simulink model "OBJMIL"  (Simulink 8.2)
settings: Solver=FixedStepDiscrete  StartTime=0.0  StopTime=126  FixedStep=0.005  RelTol=1e-3
PostLoadFcn:
  | , if any(exist('dsrtsu_mdlpostloadfcn', 'file') == [2, 3, 6]), try dsrtsu_mdlpostloadfcn('Execute', bdroot); catch fprintf('Error in PostLoadFcn (dsrtsu_mdlpostloadfcn) for model "%s":\n %s\n', bdroot, lasterr); end, end,
values from neighbouring files (symbols this model uses):
  C_TASK_5MS_S = (	C_TICK_TIME_S      	)    [hcu_local_hdr.m]
  ENUM_GEARPOSN_1ST = uint8(  1  )    [hcu_local_hdr.m]
  ENUM_GEARPOSN_R = uint8(  7  )    [hcu_local_hdr.m]
  FALSE = boolean( 0 )    [hcu_local_hdr.m]
  R_OBJ_Position = single([ii 0 0])    [GridSearch.m]
  R_OBJ_RelAccel = single([0 0 kk])    [GridSearch.m]
  R_OBJ_RelVelocity = single([0 jj 0])    [GridSearch.m]
  TRUE = boolean( 1 )    [hcu_local_hdr.m]
undefined symbols (not defined in the file or in its folder): A_OBJ, B_OBJ, C_OBJ, Gamma_OBJ, KOBJ_KalmanFilterCalRate_s, KOBJ_UseCalObjSpd_flg, KOBJ_UseEstObjInfo_flg, KOBJ_VehAccCalRate_s, KOBJ_VehAccFltConst_s, Q_OBJ, slcm
libraries: simulink x39, hcu_lib x10, dspmtrx3 x3, dspinverses x1
(part 1 of 2)
settings Model: DSRTSU_INTERNAL_RTI_VER=460  DSRTSU_INTERNAL_RTI_TYPE=rti1401  RTICANMMDATA=struct('GeneralSetupData',struct('modelroot','D:\HAITEC\SVN\trunk\ADAS_Softwares\HTDragon\software\sw_development\arch','generalsettings',struct('filesettings',struct('destfolder',struct('Name','RTICANMM_FILES','Check',1),'buildfolder',struct('Name','.','Check',1),'AbsDestfolder',struct('Name','D:\HAITEC\SVN\trunk\ADAS_Softwares\HTDragon\software\sw_development\arch\RTICANMM_FILES'),'AbsBuildfolder',struct('Name','D:\HAITEC\SVN\trunk\ADAS_Softwares\HTDragon\software\sw_development\arch'))),'options',struct('addpaths',1,'rmpaths',1,'addtrcexclusion',logical(1),'cannavigator',struct('checkmonitoring',0),'show_usrtrc',0,'use_usrtrc',0),'advanced',struct('options',[1 1 1 1 1 1 1 1 1 1 1 1 1 1 1 1 1 1 1 1 1 1 1 1 1 1 1 1 1 1 1 1 1 1 1 1 1 1 1 1 1 1 1 1 1 1 1 1 1 1 1 1 1 1 1 1 1 1 1 1 1 1 1 1 1 1 1 1 1 1 1 1 1 1 1 1 1 1 1 1 1 1 1 1 1 1 1 1 1 1 1 1 1 1 1 1 1 1 1 1]),'MPSetup',{{}},'modelname','OBJMIL','block','OBJMIL'))  DSRTSU_INTERNAL_RTIFPGA=50  Creator=14014  LastModifiedBy=14014  BufferReuse=off
settings DataIOCC: SignalLoggingSaveFormat=Dataset
settings OptimizationCC: BlockReduction=off  OptimizeBlockIOStorage=off  BufferReuse=off  ExpressionFolding=off  ExpressionDepthLimit=128  LocalBlockOutputs=off
settings DebuggingCC: ParameterPrecisionLossMsg=none  FcnCallInpInsideContextMsg=EnableAllAsError  StateNameClashWarn=none
settings HardwareCC: ProdIntDivRoundTo=Zero  ProdEndianess=BigEndian  ProdHWDeviceType=Generic->Custom  TargetIntDivRoundTo=Zero  TargetEndianess=BigEndian  TargetHWDeviceType=Generic->Custom
settings RTWCC: SystemTargetFile=rti1401.tlc  MakeCommand=make_rti  TemplateMakefile=rti1401.tmf  Description=dSPACE DS1401 Hardware Platform  ProcessScript=rti1401_make_rtw_hook
settings STFCustomTargetCC: CodeReplacementLibrary=ANSI_C  ParMdlRefBuildCompliant=on  GeneratePreprocessorConditionals=Disable all  MatFileLogging=on  SystemTargetFile=rti1401.tlc
settings GRTTargetCC: CompOptLevelCompliant=off  ConcurrentExecutionCompliant=off  ExtModeMexFile=noextcomm
settings CustomProperty: DataType=RTWOptions_EnumType_C__Program Files_dSPACE RCPHIL 2015-A_MATLAB_RTI_RTI1401_TLC_rti1401_1InitialSimState  Value=RUN
settings EnumStrPairs: String=RUN

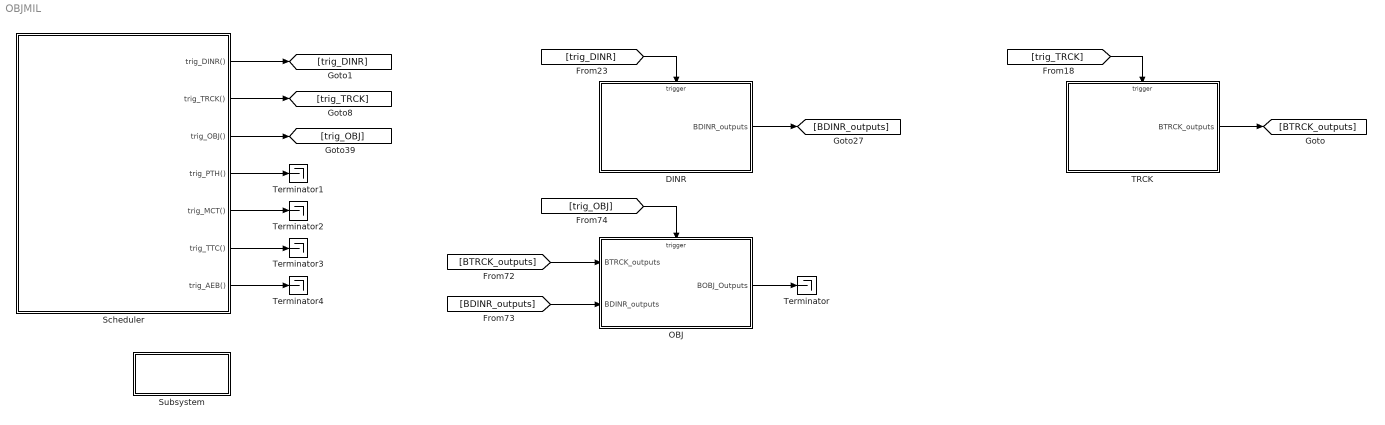
== system OBJMIL ==
  DINR : Subsystem
      settings: RTWSystemCode=Nonreusable function  RTWFcnNameOpts=Use subsystem name  RTWFileNameOpts=Use subsystem name
  OBJ : Subsystem
      settings: RTWSystemCode=Nonreusable function  RTWFcnNameOpts=Use subsystem name  RTWFileNameOpts=Use subsystem name
  Scheduler : Stateflow chart  TreatAsAtomicUnit=on
  Subsystem : Subsystem
      settings: OpenFcn=load AEBMIL_Data.mat;
      mask Display: disp('Double-Click\nTo Load Data')
  TRCK : Subsystem
      settings: RTWSystemCode=Nonreusable function  RTWFcnNameOpts=Use subsystem name  RTWFileNameOpts=Use subsystem name
  Terminator{,1..4} (5 alike) : Terminator
  wires:
  Scheduler/4(trig_PTH()) -> Terminator1/1
  Scheduler/6(trig_TTC()) -> Terminator3/1
  Scheduler/7(trig_AEB()) -> Terminator4/1
  [BTRCK_outputs] -> OBJ/1(BTRCK_outputs)
  [BDINR_outputs] -> OBJ/2(BDINR_outputs)
  OBJ/1(BOBJ_Outputs) -> Terminator/1
  [trig_OBJ] -> OBJ/Trigger
  Scheduler/3(trig_OBJ()) -> [trig_OBJ]
  Scheduler/5(trig_MCT()) -> Terminator2/1
  [trig_DINR] -> DINR/Trigger
  DINR/1(BDINR_outputs) -> [BDINR_outputs]
  Scheduler/1(trig_DINR()) -> [trig_DINR]
  TRCK/1(BTRCK_outputs) -> [BTRCK_outputs]
  [trig_TRCK] -> TRCK/Trigger
  Scheduler/2(trig_TRCK()) -> [trig_TRCK]

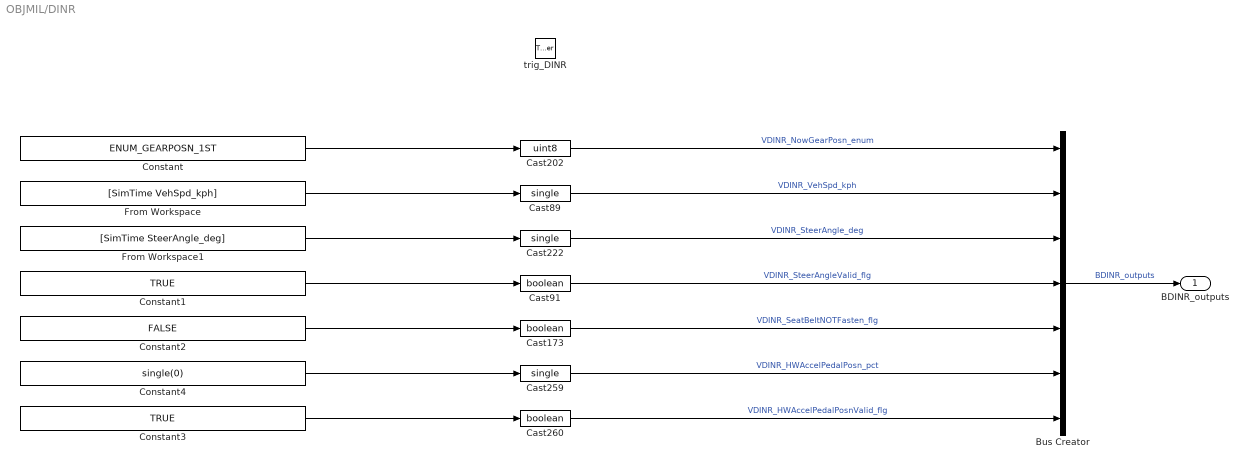
== system OBJMIL/DINR ==
  trig_DINR : TriggerPort  TriggerType=function-call
  Bus Creator : BusCreator  Inputs=7
  Cast173 : DataTypeConversion  OutDataTypeStr=boolean  RndMeth=Zero
  Cast202 : DataTypeConversion  OutDataTypeStr=uint8  RndMeth=Zero
  Cast222 : DataTypeConversion  OutDataTypeStr=single  RndMeth=Zero
  Cast259 : DataTypeConversion  OutDataTypeStr=single  RndMeth=Zero
  Cast260 : DataTypeConversion  OutDataTypeStr=boolean  RndMeth=Zero
  Cast89 : DataTypeConversion  OutDataTypeStr=single  RndMeth=Zero
  Cast91 : DataTypeConversion  OutDataTypeStr=boolean  RndMeth=Zero
  Constant : Constant  Value=ENUM_GEARPOSN_1ST
  Constant1 : Constant  Value=TRUE
  Constant2 : Constant  Value=FALSE
  Constant3 : Constant  Value=TRUE
  Constant4 : Constant  Value=single(0)
  From Workspace : FromWorkspace  VariableName=[SimTime VehSpd_kph]  Interpolate=off  OutputAfterFinalValue=Setting to zero
  From Workspace1 : FromWorkspace  VariableName=[SimTime SteerAngle_deg]  Interpolate=off  OutputAfterFinalValue=Setting to zero
  BDINR_outputs : Outport
  wires:
  Constant3/1 -> Cast260/1
  Constant4/1 -> Cast259/1
  Constant2/1 -> Cast173/1
  From Workspace1/1 -> Cast222/1
  Constant1/1 -> Cast91/1
  From Workspace/1 -> Cast89/1
  Constant/1 -> Cast202/1
  Cast260/1 -> Bus Creator/7  "VDINR_HWAccelPedalPosnValid_flg"
  Cast259/1 -> Bus Creator/6  "VDINR_HWAccelPedalPosn_pct"
  Cast173/1 -> Bus Creator/5  "VDINR_SeatBeltNOTFasten_flg"
  Cast202/1 -> Bus Creator/1  "VDINR_NowGearPosn_enum"
  Cast222/1 -> Bus Creator/3  "VDINR_SteerAngle_deg"
  Cast91/1 -> Bus Creator/4  "VDINR_SteerAngleValid_flg"
  Cast89/1 -> Bus Creator/2  "VDINR_VehSpd_kph"
  Bus Creator/1 -> BDINR_outputs/1  "BDINR_outputs"

== system OBJMIL/OBJ ==
  BTRCK_outputs : Inport  OutDataTypeStr=Bus: BTRCK_outputs
  BDINR_outputs : Inport  Port=2
  trig_OBJ : TriggerPort  TriggerType=function-call
  Bus Creator : BusCreator  Inputs=20  OutDataTypeStr=Bus: BOBJ_outputs
  Bus Selector3 : BusSelector  OutputSignals=VTRCK_Obj1PositionX_m,VTRCK_Obj1RelVelocityX_mps,VTRCK_Obj1Valid_flg,VTRCK_Obj1ConfidLevel_enum,VTRCK_Obj2PositionX_m,VTRCK_Obj2RelVelocityX_mps,VTRCK_Obj2Valid_flg,VTRCK_Obj2ConfidLevel_enum,VTRCK_Obj3PositionX_m,VTRCK_Obj3RelVelocityX_mps,VTRCK_Obj3Valid_flg,VTRCK_Obj3ConfidLevel_enum,VTRCK_Obj4PositionX_m,VTRCK_Obj4RelVelocityX_mps,VTRCK_Obj4Valid_flg,VTRCK_Obj4ConfidLevel_enum,VTRCK_Obj5PositionX_m,VTRCK_Obj5RelVelocityX_mps,VTRCK_Obj5Valid_flg,VTRCK_Obj5ConfidLevel_enum
  Bus Selector5 : BusSelector  OutputSignals=VDINR_VehSpd_kph,VDINR_NowGearPosn_enum
  OBJ : Subsystem
  model_info : Subsystem  LoadFcn=slcm LoadBlock;  InitFcn=slcm('UpdateAllCMBlocksInThisModelInit')  mask(CMBlock){InitialSaveTempField=, InitialBlockCM=None, BlockCM=None, Frame=on, SaveTempField=, DisplayStringWithTags=$Id: ttc.mdl 800 2014-08-28 03:32:11Z JuneXmas $, MaskDisplayString=$Id: ttc.mdl 800 2014-08-28 03:32:11Z JuneXmas $, HorizontalTextAlignment=Center, LeftAlignmentValue=0.5, SourceBlockDiagram=OBJMIL, TagMaxNumber=20, CMTag1=, CMTag2=, CMTag3=, CMTag4=, CMTag5=, CMTag6=, CMTag7=, CMTag8=, CMTag9=, CMTag10=, CMTag11=, CMTag12=, CMTag13=, CMTag14=, CMTag15=, CMTag16=, CMTag17=, CMTag18=, CMTag19=, CMTag20=}
      mask help: This block allows revision control information to be displayed within the model.
      settings: CopyFcn=slcm CopyBlock;  DeleteFcn=slcm Cancel;  PostSaveFcn=slcm('UpdateAllCMBlocksInThisModel')  NameChangeFcn=slcm Rename;  OpenFcn=slcm
      mask Display: text(str2num(LeftAlignmentValue), 0.5, MaskDisplayString, 'HorizontalAlignment', HorizontalTextAlignment)
  BOBJ_Outputs : Outport  OutDataTypeStr=Bus: BOBJ_outputs
  wires:
  Bus Creator/1 -> BOBJ_Outputs/1  "BOBJ_outputs"
  BTRCK_outputs/1 -> Bus Selector3/1
  Bus Selector3/14 -> OBJ/14(VTRCK_Obj4RelVelocityX_mps)  "<VTRCK_Obj4RelVelocityX_mps>"
  Bus Selector3/10 -> OBJ/10(VTRCK_Obj3RelVelocityX_mps)  "<VTRCK_Obj3RelVelocityX_mps>"
  Bus Selector3/9 -> OBJ/9(VTRCK_Obj3PositionX_m)  "<VTRCK_Obj3PositionX_m>"
  Bus Selector3/2 -> OBJ/2(VTRCK_Obj1RelVelocityX_mps)  "<VTRCK_Obj1RelVelocityX_mps>"
  Bus Selector3/6 -> OBJ/6(VTRCK_Obj2RelVelocityX_mps)  "<VTRCK_Obj2RelVelocityX_mps>"
  Bus Selector3/18 -> OBJ/18(VTRCK_Obj5RelVelocityX_mps)  "<VTRCK_Obj5RelVelocityX_mps>"
  Bus Selector3/1 -> OBJ/1(VTRCK_Obj1PositionX_m)  "<VTRCK_Obj1PositionX_m>"
  Bus Selector3/5 -> OBJ/5(VTRCK_Obj2PositionX_m)  "<VTRCK_Obj2PositionX_m>"
  Bus Selector3/13 -> OBJ/13(VTRCK_Obj4PositionX_m)  "<VTRCK_Obj4PositionX_m>"
  Bus Selector3/17 -> OBJ/17(VTRCK_Obj5PositionX_m)  "<VTRCK_Obj5PositionX_m>"
  Bus Selector5/1 -> OBJ/21(VDINR_VehSpd_kph)  "<VDINR_VehSpd_kph>"
  BDINR_outputs/1 -> Bus Selector5/1
  Bus Selector3/3 -> OBJ/3(VTRCK_Obj1Valid_flg)  "<VTRCK_Obj1Valid_flg>"
  Bus Selector3/7 -> OBJ/7(VTRCK_Obj2Valid_flg)  "<VTRCK_Obj2Valid_flg>"
  Bus Selector3/11 -> OBJ/11(VTRCK_Obj3Valid_flg)  "<VTRCK_Obj3Valid_flg>"
  Bus Selector3/15 -> OBJ/15(VTRCK_Obj4Valid_flg)  "<VTRCK_Obj4Valid_flg>"
  Bus Selector3/19 -> OBJ/19(VTRCK_Obj5Valid_flg)  "<VTRCK_Obj5Valid_flg>"
  OBJ/1(VOBJ_Obj1PositionX_m) -> Bus Creator/1
  OBJ/2(VOBJ_Obj1RelVelocityX_mps) -> Bus Creator/2
  OBJ/3(VOBJ_Obj1RelAccX_mps2) -> Bus Creator/3
  OBJ/4(VOBJ_Obj1Valid_flg) -> Bus Creator/4
  OBJ/5(VOBJ_Obj2PositionX_m) -> Bus Creator/5
  OBJ/6(VOBJ_Obj2RelVelocityX_mps) -> Bus Creator/6
  OBJ/7(VOBJ_Obj2RelAccX_mps2) -> Bus Creator/7
  OBJ/8(VOBJ_Obj2Valid_flg) -> Bus Creator/8
  OBJ/9(VOBJ_Obj3PositionX_m) -> Bus Creator/9
  OBJ/10(VOBJ_Obj3RelVelocityX_mps) -> Bus Creator/10
  OBJ/11(VOBJ_Obj3RelAccX_mps2) -> Bus Creator/11
  OBJ/12(VOBJ_Obj3Valid_flg) -> Bus Creator/12
  OBJ/13(VOBJ_Obj4PositionX_m) -> Bus Creator/13
  OBJ/14(VOBJ_Obj4RelVelocityX_mps) -> Bus Creator/14
  OBJ/15(VOBJ_Obj4RelAccX_mps2) -> Bus Creator/15
  OBJ/16(VOBJ_Obj4Valid_flg) -> Bus Creator/16
  OBJ/17(VOBJ_Obj5PositionX_m) -> Bus Creator/17
  OBJ/18(VOBJ_Obj5RelVelocityX_mps) -> Bus Creator/18
  OBJ/19(VOBJ_Obj5RelAccX_mps2) -> Bus Creator/19
  OBJ/20(VOBJ_Obj5Valid_flg) -> Bus Creator/20
  Bus Selector5/2 -> OBJ/22(VDINR_NowGearPosn_enum)  "<VDINR_NowGearPosn_enum>"
  Bus Selector3/4 -> OBJ/4(VTRCK_Obj1ConfidLevel_enum)  "<VTRCK_Obj1ConfidLevel_enum>"
  Bus Selector3/8 -> OBJ/8(VTRCK_Obj2ConfidLevel_enum)  "<VTRCK_Obj2ConfidLevel_enum>"
  Bus Selector3/12 -> OBJ/12(VTRCK_Obj3ConfidLevel_enum)  "<VTRCK_Obj3ConfidLevel_enum>"
  Bus Selector3/16 -> OBJ/16(VTRCK_Obj4ConfidLevel_enum)  "<VTRCK_Obj4ConfidLevel_enum>"
  Bus Selector3/20 -> OBJ/20(VTRCK_Obj5ConfidLevel_enum)  "<VTRCK_Obj5ConfidLevel_enum>"

== system OBJMIL/Subsystem ==

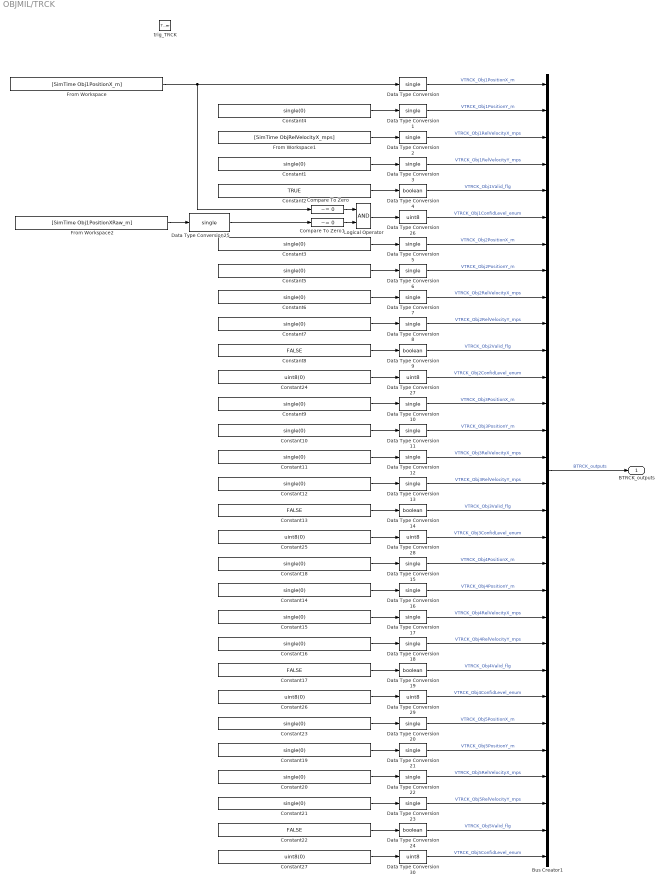
== system OBJMIL/TRCK ==
  trig_TRCK : TriggerPort  TriggerType=function-call
  Bus Creator1 : BusCreator  Inputs=30  OutDataTypeStr=Bus: BTRCK_outputs
  Compare To Zero : simulink/Logic and Bit Operations/Compare To Zero  relop=~=  OutDataTypeStr=boolean
  Compare To Zero1 : simulink/Logic and Bit Operations/Compare To Zero  relop=~=  OutDataTypeStr=boolean
  Constant{1,3..7,9..12,14..16,18..21,23} (18 alike) : Constant  Value=single(0)
  Constant{8,13,17,22} (4 alike) : Constant  Value=FALSE
  Constant2 : Constant  Value=TRUE
  Constant{24..27} (4 alike) : Constant  Value=uint8(0)
  Data Type Conversion{,1..3,5..8,10..13,15..18,20..23,25} (21 alike) : DataTypeConversion  OutDataTypeStr=single
  Data Type Conversion{4,9,14,19,24} (5 alike) : DataTypeConversion  OutDataTypeStr=boolean
  Data Type Conversion{26..30} (5 alike) : DataTypeConversion  OutDataTypeStr=uint8
  From Workspace : FromWorkspace  VariableName=[SimTime Obj1PositionX_m]  Interpolate=off  OutputAfterFinalValue=Setting to zero
  From Workspace1 : FromWorkspace  VariableName=[SimTime ObjRelVelocityX_mps]  Interpolate=off  OutputAfterFinalValue=Setting to zero
  From Workspace2 : FromWorkspace  VariableName=[SimTime Obj1PositionXRaw_m]  Interpolate=off  OutputAfterFinalValue=Setting to zero
  Logical Operator : Logic  AllPortsSameDT=off  OutDataTypeStr=boolean
  BTRCK_outputs : Outport  OutDataTypeStr=Bus: BTRCK_outputs
  wires:
  Bus Creator1/1 -> BTRCK_outputs/1  "BTRCK_outputs"
  Constant4/1 -> Data Type Conversion1/1
  From Workspace1/1 -> Data Type Conversion2/1
  Constant1/1 -> Data Type Conversion3/1
  Constant3/1 -> Data Type Conversion5/1
  Constant5/1 -> Data Type Conversion6/1
  Constant6/1 -> Data Type Conversion7/1
  Constant7/1 -> Data Type Conversion8/1
  Constant9/1 -> Data Type Conversion10/1
  Constant10/1 -> Data Type Conversion11/1
  Constant11/1 -> Data Type Conversion12/1
  Constant12/1 -> Data Type Conversion13/1
  Constant18/1 -> Data Type Conversion15/1
  Constant14/1 -> Data Type Conversion16/1
  Constant15/1 -> Data Type Conversion17/1
  Constant16/1 -> Data Type Conversion18/1
  Constant23/1 -> Data Type Conversion20/1
  Constant19/1 -> Data Type Conversion21/1
  Constant20/1 -> Data Type Conversion22/1
  Constant21/1 -> Data Type Conversion23/1
  Data Type Conversion3/1 -> Bus Creator1/4  "VTRCK_Obj1RelVelocityY_mps"
  Data Type Conversion1/1 -> Bus Creator1/2  "VTRCK_Obj1PositionY_m"
  Data Type Conversion2/1 -> Bus Creator1/3  "VTRCK_Obj1RelVelocityX_mps"
  Data Type Conversion/1 -> Bus Creator1/1  "VTRCK_Obj1PositionX_m"
  Data Type Conversion15/1 -> Bus Creator1/19  "VTRCK_Obj4PositionX_m"
  Data Type Conversion18/1 -> Bus Creator1/22  "VTRCK_Obj4RelVelocityY_mps"
  Data Type Conversion17/1 -> Bus Creator1/21  "VTRCK_Obj4RelVelocityX_mps"
  Data Type Conversion16/1 -> Bus Creator1/20  "VTRCK_Obj4PositionY_m"
  Data Type Conversion22/1 -> Bus Creator1/27  "VTRCK_Obj5RelVelocityX_mps"
  Data Type Conversion19/1 -> Bus Creator1/23  "VTRCK_Obj4Valid_flg"
  Data Type Conversion4/1 -> Bus Creator1/5  "VTRCK_Obj1Valid_flg"
  Data Type Conversion8/1 -> Bus Creator1/10  "VTRCK_Obj2RelVelocityY_mps"
  Data Type Conversion5/1 -> Bus Creator1/7  "VTRCK_Obj2PositionX_m"
  Data Type Conversion6/1 -> Bus Creator1/8  "VTRCK_Obj2PositionY_m"
  Data Type Conversion9/1 -> Bus Creator1/11  "VTRCK_Obj2Valid_flg"
  Data Type Conversion7/1 -> Bus Creator1/9  "VTRCK_Obj2RelVelocityX_mps"
  Data Type Conversion11/1 -> Bus Creator1/14  "VTRCK_Obj3PositionY_m"
  Data Type Conversion12/1 -> Bus Creator1/15  "VTRCK_Obj3RelVelocityX_mps"
  Data Type Conversion13/1 -> Bus Creator1/16  "VTRCK_Obj3RelVelocityY_mps"
  Data Type Conversion14/1 -> Bus Creator1/17  "VTRCK_Obj3Valid_flg"
  Data Type Conversion10/1 -> Bus Creator1/13  "VTRCK_Obj3PositionX_m"
  Data Type Conversion20/1 -> Bus Creator1/25  "VTRCK_Obj5PositionX_m"
  Data Type Conversion21/1 -> Bus Creator1/26  "VTRCK_Obj5PositionY_m"
  Data Type Conversion24/1 -> Bus Creator1/29  "VTRCK_Obj5Valid_flg"
  Data Type Conversion23/1 -> Bus Creator1/28  "VTRCK_Obj5RelVelocityY_mps"
  Constant2/1 -> Data Type Conversion4/1
  Constant8/1 -> Data Type Conversion9/1
  Constant13/1 -> Data Type Conversion14/1
  Constant17/1 -> Data Type Conversion19/1
  Constant22/1 -> Data Type Conversion24/1
  Logical Operator/1 -> Data Type Conversion26/1
  Data Type Conversion26/1 -> Bus Creator1/6  "VTRCK_Obj1ConfidLevel_enum"
  Data Type Conversion27/1 -> Bus Creator1/12  "VTRCK_Obj2ConfidLevel_enum"
  Constant24/1 -> Data Type Conversion27/1
  Data Type Conversion28/1 -> Bus Creator1/18  "VTRCK_Obj3ConfidLevel_enum"
  Constant25/1 -> Data Type Conversion28/1
  Data Type Conversion29/1 -> Bus Creator1/24  "VTRCK_Obj4ConfidLevel_enum"
  Constant26/1 -> Data Type Conversion29/1
  Data Type Conversion30/1 -> Bus Creator1/30  "VTRCK_Obj5ConfidLevel_enum"
  Constant27/1 -> Data Type Conversion30/1
  Compare To Zero1/1 -> Logical Operator/2
  Compare To Zero/1 -> Logical Operator/1
  Data Type Conversion25/1 -> Compare To Zero1/1
  From Workspace2/1 -> Data Type Conversion25/1
  From Workspace/1 -> Compare To Zero/1, Data Type Conversion/1

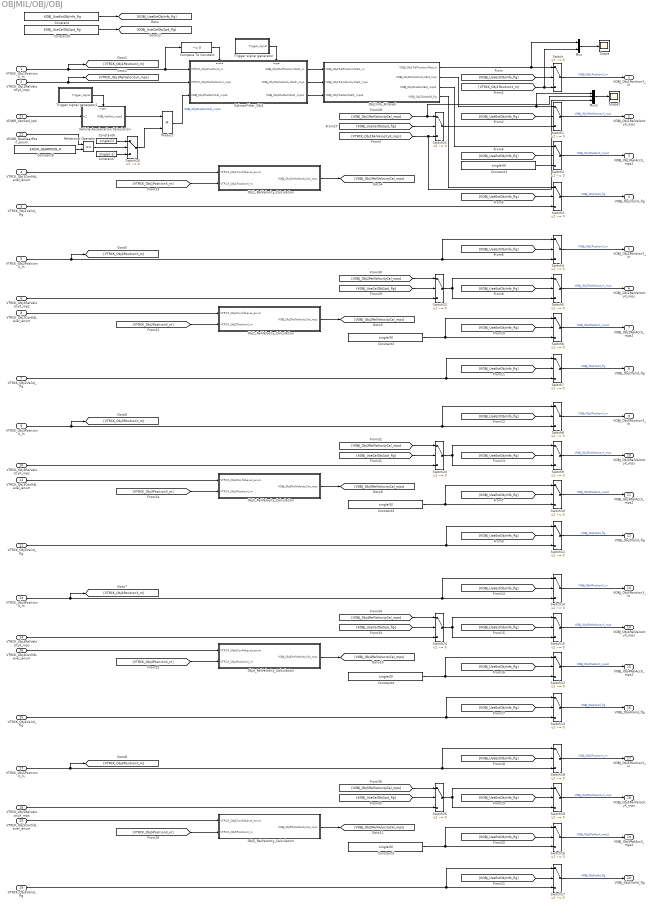
== system OBJMIL/OBJ/OBJ ==
  VTRCK_Obj1PositionX_m : Inport
  VTRCK_Obj1RelVelocityX_mps : Inport  Port=2
  VTRCK_Obj1Valid_flg : Inport  Port=3
  VTRCK_Obj1ConfidLevel_enum : Inport  Port=4
  VTRCK_Obj2PositionX_m : Inport  Port=5
  VTRCK_Obj2RelVelocityX_mps : Inport  Port=6
  VTRCK_Obj2Valid_flg : Inport  Port=7
  VTRCK_Obj2ConfidLevel_enum : Inport  Port=8
  VTRCK_Obj3PositionX_m : Inport  Port=9
  VTRCK_Obj3RelVelocityX_mps : Inport  Port=10
  VTRCK_Obj3Valid_flg : Inport  Port=11
  VTRCK_Obj3ConfidLevel_enum : Inport  Port=12
  VTRCK_Obj4PositionX_m : Inport  Port=13
  VTRCK_Obj4RelVelocityX_mps : Inport  Port=14
  VTRCK_Obj4Valid_flg : Inport  Port=15
  VTRCK_Obj4ConfidLevel_enum : Inport  Port=16
  VTRCK_Obj5PositionX_m : Inport  Port=17
  VTRCK_Obj5RelVelocityX_mps : Inport  Port=18
  VTRCK_Obj5Valid_flg : Inport  Port=19
  VTRCK_Obj5ConfidLevel_enum : Inport  Port=20
  VDINR_VehSpd_kph : Inport  Port=21
  VDINR_NowGearPosn_enum : Inport  Port=22
  Compare To Constant : simulink/Logic and Bit Operations/Compare To Constant  relop=~=  const=0  OutDataTypeStr=boolean
  Constant : Constant  Value=KOBJ_UseEstObjInfo_flg
  Constant{1..5} (5 alike) : Constant  Value=single(0)
  Constant6 : Constant  Value=single(1)
  Constant7 : Constant  Value=single(-1)
  Constant8 : Constant  Value=ENUM_GEARPOSN_R
  Constant9 : Constant  Value=KOBJ_UseCalObjSpd_flg
  KalmanFilter_Obj1 : Subsystem
  Mux : Mux  Inputs=2
  Mux1 : Mux  Inputs=3
  Obj1Info_Filtered : Subsystem
  Obj1_RelVelocity_Calculation : Subsystem
  Obj2_RelVelocity_Calculation : Subsystem
  Obj3_RelVelocity_Calculation : Subsystem
  Obj4_RelVelocity_Calculation : Subsystem
  Obj5_RelVelocity_Calculation : Subsystem
  Product : Product
  Relational Operator : RelationalOperator  Operator===  OutDataTypeStr=boolean
  Scope : Scope
  Scope1 : Scope
  Switch{,1..25} (26 alike) : Switch  Criteria=u2 ~= 0
  Trigger signal generator : Subsystem  TreatAsAtomicUnit=on
  Trigger signal generator1 : Subsystem  TreatAsAtomicUnit=on
  Vehicle Acceleration Calculation : Subsystem
  VOBJ_Obj1PositionX_m : Outport
  VOBJ_Obj1RelVelocityX_mps : Outport  Port=2
  VOBJ_Obj1RelAccX_mps2 : Outport  Port=3
  VOBJ_Obj1Valid_flg : Outport  Port=4
  VOBJ_Obj2PositionX_m : Outport  Port=5
  VOBJ_Obj2RelVelocityX_mps : Outport  Port=6
  VOBJ_Obj2RelAccX_mps2 : Outport  Port=7
  VOBJ_Obj2Valid_flg : Outport  Port=8
  VOBJ_Obj3PositionX_m : Outport  Port=9
  VOBJ_Obj3RelVelocityX_mps : Outport  Port=10
  VOBJ_Obj3RelAccX_mps2 : Outport  Port=11
  VOBJ_Obj3Valid_flg : Outport  Port=12
  VOBJ_Obj4PositionX_m : Outport  Port=13
  VOBJ_Obj4RelVelocityX_mps : Outport  Port=14
  VOBJ_Obj4RelAccX_mps2 : Outport  Port=15
  VOBJ_Obj4Valid_flg : Outport  Port=16
  VOBJ_Obj5PositionX_m : Outport  Port=17
  VOBJ_Obj5RelVelocityX_mps : Outport  Port=18
  VOBJ_Obj5RelAccX_mps2 : Outport  Port=19
  VOBJ_Obj5Valid_flg : Outport  Port=20
  wires:
  Trigger signal generator/1(Trigger_signal) -> KalmanFilter_Obj1/Trigger
  VTRCK_Obj1PositionX_m/1 -> KalmanFilter_Obj1/1(VTRCK_Obj1PositionX_m), Compare To Constant/1, [VTRCK_Obj1PositionX_m]
  VTRCK_Obj1RelVelocityX_mps/1 -> [VTRCK_Obj1RelVelocityX_mps], KalmanFilter_Obj1/2(VTRCK_Obj1RelVelocityX_mps)
  Compare To Constant/1 -> KalmanFilter_Obj1/Enable
  Trigger signal generator1/1(Trigger_signal) -> Vehicle Acceleration Calculation/Trigger
  VDINR_VehSpd_kph/1 -> Vehicle Acceleration Calculation/1(In1)
  Vehicle Acceleration Calculation/1(VOBJ_VehAcc_mps2) -> Product/1
  Product/1 -> KalmanFilter_Obj1/3(VOBJ_Obj1RelAccXCal_mps2)  "VOBJ_Obj1RelAccXCal_mps2"
  KalmanFilter_Obj1/1(VOBJ_Obj1RelPositionXKalF_m) -> Obj1Info_Filtered/1(VOBJ_Obj1RelPositionXKalF_m)
  KalmanFilter_Obj1/2(VOBJ_Obj1RelVelocityXKalF_mps) -> Obj1Info_Filtered/2(VOBJ_Obj1RelVelocityXKalF_mps)
  KalmanFilter_Obj1/3(VOBJ_Obj1RelAccXKalF_mps2) -> Obj1Info_Filtered/3(VOBJ_Obj1RelAccXKalF_mps2)
  VTRCK_Obj1Valid_flg/1 -> Switch3/3
  Constant/1 -> [KOBJ_UseEstObjInfo_flg]
  [KOBJ_UseEstObjInfo_flg] -> Switch/2
  Switch/1 -> VOBJ_Obj1PositionX_m/1  "VOBJ_Obj1PositionX_m"
  [VTRCK_Obj1PositionX_m] -> Mux/2, Switch/3
  Obj1Info_Filtered/1(VOBJ_Obj1RelPositionXEst_m) -> Mux/1, Switch/1
  [KOBJ_UseEstObjInfo_flg] -> Switch1/2
  Switch1/1 -> VOBJ_Obj1RelVelocityX_mps/1  "VOBJ_Obj1RelVelocityX_mps"
  Obj1Info_Filtered/2(VOBJ_Obj1RelVelocityXEst_mps) -> Mux1/1, Switch1/1
  [KOBJ_UseEstObjInfo_flg] -> Switch2/2
  Constant1/1 -> Switch2/3
  Obj1Info_Filtered/3(VOBJ_Obj1RelAccXEst_mps2) -> Switch2/1
  Switch2/1 -> VOBJ_Obj1RelAccX_mps2/1  "VOBJ_Obj1RelAccX_mps2"
  [KOBJ_UseEstObjInfo_flg] -> Switch3/2
  Switch3/1 -> VOBJ_Obj1Valid_flg/1  "VOBJ_Obj1Valid_flg"
  Obj1Info_Filtered/4(VOBJ_Obj1EstValid_flg) -> Switch3/1
  VTRCK_Obj2Valid_flg/1 -> Switch7/1, Switch7/3
  [KOBJ_UseEstObjInfo_flg] -> Switch4/2
  Switch4/1 -> VOBJ_Obj2PositionX_m/1  "VOBJ_Obj2PositionX_m"
  VTRCK_Obj2PositionX_m/1 -> [VTRCK_Obj2PositionX_m], Switch4/1, Switch4/3
  [KOBJ_UseEstObjInfo_flg] -> Switch5/2
  Switch5/1 -> VOBJ_Obj2RelVelocityX_mps/1  "VOBJ_Obj2RelVelocityX_mps"
  [KOBJ_UseEstObjInfo_flg] -> Switch6/2
  Constant2/1 -> Switch6/1, Switch6/3
  Switch6/1 -> VOBJ_Obj2RelAccX_mps2/1  "VOBJ_Obj2RelAccX_mps2"
  [KOBJ_UseEstObjInfo_flg] -> Switch7/2
  Switch7/1 -> VOBJ_Obj2Valid_flg/1  "VOBJ_Obj2Valid_flg"
  VTRCK_Obj3Valid_flg/1 -> Switch11/3, Switch11/1
  [KOBJ_UseEstObjInfo_flg] -> Switch8/2
  Switch8/1 -> VOBJ_Obj3PositionX_m/1  "VOBJ_Obj3PositionX_m"
  VTRCK_Obj3PositionX_m/1 -> [VTRCK_Obj3PositionX_m], Switch8/3, Switch8/1
  [KOBJ_UseEstObjInfo_flg] -> Switch9/2
  Switch9/1 -> VOBJ_Obj3RelVelocityX_mps/1  "VOBJ_Obj3RelVelocityX_mps"
  VTRCK_Obj3RelVelocityX_mps/1 -> Switch23/3
  [KOBJ_UseEstObjInfo_flg] -> Switch10/2
  Constant3/1 -> Switch10/3, Switch10/1
  Switch10/1 -> VOBJ_Obj3RelAccX_mps2/1  "VOBJ_Obj3RelAccX_mps2"
  [KOBJ_UseEstObjInfo_flg] -> Switch11/2
  Switch11/1 -> VOBJ_Obj3Valid_flg/1  "VOBJ_Obj3Valid_flg"
  VTRCK_Obj4Valid_flg/1 -> Switch13/1, Switch13/3
  [KOBJ_UseEstObjInfo_flg] -> Switch14/2
  Switch14/1 -> VOBJ_Obj4PositionX_m/1  "VOBJ_Obj4PositionX_m"
  VTRCK_Obj4PositionX_m/1 -> [VTRCK_Obj4PositionX_m], Switch14/1, Switch14/3
  [KOBJ_UseEstObjInfo_flg] -> Switch15/2
  Switch15/1 -> VOBJ_Obj4RelVelocityX_mps/1  "VOBJ_Obj4RelVelocityX_mps"
  VTRCK_Obj4RelVelocityX_mps/1 -> Switch24/3
  [KOBJ_UseEstObjInfo_flg] -> Switch12/2
  Constant4/1 -> Switch12/1, Switch12/3
  Switch12/1 -> VOBJ_Obj4RelAccX_mps2/1  "VOBJ_Obj4RelAccX_mps2"
  [KOBJ_UseEstObjInfo_flg] -> Switch13/2
  Switch13/1 -> VOBJ_Obj4Valid_flg/1  "VOBJ_Obj4Valid_flg"
  VTRCK_Obj5Valid_flg/1 -> Switch17/3, Switch17/1
  [KOBJ_UseEstObjInfo_flg] -> Switch18/2
  Switch18/1 -> VOBJ_Obj5PositionX_m/1  "VOBJ_Obj5PositionX_m"
  VTRCK_Obj5PositionX_m/1 -> [VTRCK_Obj5PositionX_m], Switch18/3, Switch18/1
  [KOBJ_UseEstObjInfo_flg] -> Switch19/2
  Switch19/1 -> VOBJ_Obj5RelVelocityX_mps/1  "VOBJ_Obj5RelVelocityX_mps"
  VTRCK_Obj5RelVelocityX_mps/1 -> Switch25/3
  [KOBJ_UseEstObjInfo_flg] -> Switch16/2
  Constant5/1 -> Switch16/3, Switch16/1
  Switch16/1 -> VOBJ_Obj5RelAccX_mps2/1  "VOBJ_Obj5RelAccX_mps2"
  [KOBJ_UseEstObjInfo_flg] -> Switch17/2
  Switch17/1 -> VOBJ_Obj5Valid_flg/1  "VOBJ_Obj5Valid_flg"
  VDINR_NowGearPosn_enum/1 -> Relational Operator/1
  Constant8/1 -> Relational Operator/2
  Relational Operator/1 -> Switch20/2
  Constant6/1 -> Switch20/1
  Constant7/1 -> Switch20/3
  Switch20/1 -> Product/2
  VTRCK_Obj5ConfidLevel_enum/1 -> Obj5_RelVelocity_Calculation/1(VTRCK_Obj5ConfidLevel_enum)
  [VTRCK_Obj5PositionX_m] -> Obj5_RelVelocity_Calculation/2(VTRCK_Obj5PositionX_m)
  Obj5_RelVelocity_Calculation/1(VOBJ_Obj5RelVelocityCal_mps) -> [VOBJ_Obj5RelVelocityCal_mps]
  VTRCK_Obj4ConfidLevel_enum/1 -> Obj4_RelVelocity_Calculation/1(VTRCK_Obj4ConfidLevel_enum)
  [VTRCK_Obj4PositionX_m] -> Obj4_RelVelocity_Calculation/2(VTRCK_Obj4PositionX_m)
  Obj4_RelVelocity_Calculation/1(VOBJ_Obj4RelVelocityCal_mps) -> [VOBJ_Obj4RelVelocityCal_mps]
  VTRCK_Obj3ConfidLevel_enum/1 -> Obj3_RelVelocity_Calculation/1(VTRCK_Obj3ConfidLevel_enum)
  [VTRCK_Obj3PositionX_m] -> Obj3_RelVelocity_Calculation/2(VTRCK_Obj3PositionX_m)
  Obj3_RelVelocity_Calculation/1(VOBJ_Obj3RelVelocityCal_mps) -> [VOBJ_Obj3RelVelocityCal_mps]
  VTRCK_Obj2ConfidLevel_enum/1 -> Obj2_RelVelocity_Calculation/1(VTRCK_Obj2ConfidLevel_enum)
  [VTRCK_Obj2PositionX_m] -> Obj2_RelVelocity_Calculation/2(VTRCK_Obj2PositionX_m)
  Obj2_RelVelocity_Calculation/1(VOBJ_Obj2RelVelocityCal_mps) -> [VOBJ_Obj2RelVelocityCal_mps]
  VTRCK_Obj1ConfidLevel_enum/1 -> Obj1_RelVelocity_Calculation/1(VTRCK_Obj1ConfidLevel_enum)
  [VTRCK_Obj1PositionX_m] -> Obj1_RelVelocity_Calculation/2(VTRCK_Obj1PositionX_m)
  Obj1_RelVelocity_Calculation/1(VOBJ_Obj1RelVelocityCal_mps) -> [VOBJ_Obj1RelVelocityCal_mps]
  Constant9/1 -> [KOBJ_UseCalObjSpd_flg]
  [KOBJ_UseCalObjSpd_flg] -> Switch21/2
  [VOBJ_Obj1RelVelocityCal_mps] -> Mux1/2, Switch21/1
  [VTRCK_Obj1RelVelocityX_mps] -> Mux1/3, Switch21/3
  Switch21/1 -> Switch1/3
  [KOBJ_UseCalObjSpd_flg] -> Switch22/2
  [VOBJ_Obj2RelVelocityCal_mps] -> Switch22/1
  VTRCK_Obj2RelVelocityX_mps/1 -> Switch22/3
  Switch22/1 -> Switch5/3, Switch5/1
  [KOBJ_UseCalObjSpd_flg] -> Switch23/2
  [VOBJ_Obj3RelVelocityCal_mps] -> Switch23/1
  Switch23/1 -> Switch9/1, Switch9/3
  [KOBJ_UseCalObjSpd_flg] -> Switch24/2
  [VOBJ_Obj4RelVelocityCal_mps] -> Switch24/1
  Switch24/1 -> Switch15/1, Switch15/3
  [KOBJ_UseCalObjSpd_flg] -> Switch25/2
  [VOBJ_Obj5RelVelocityCal_mps] -> Switch25/1
  Switch25/1 -> Switch19/1, Switch19/3
  Mux/1 -> Scope/1
  Mux1/1 -> Scope1/1

== system OBJMIL/OBJ/model_info ==
  EmptySubsystem : Subsystem

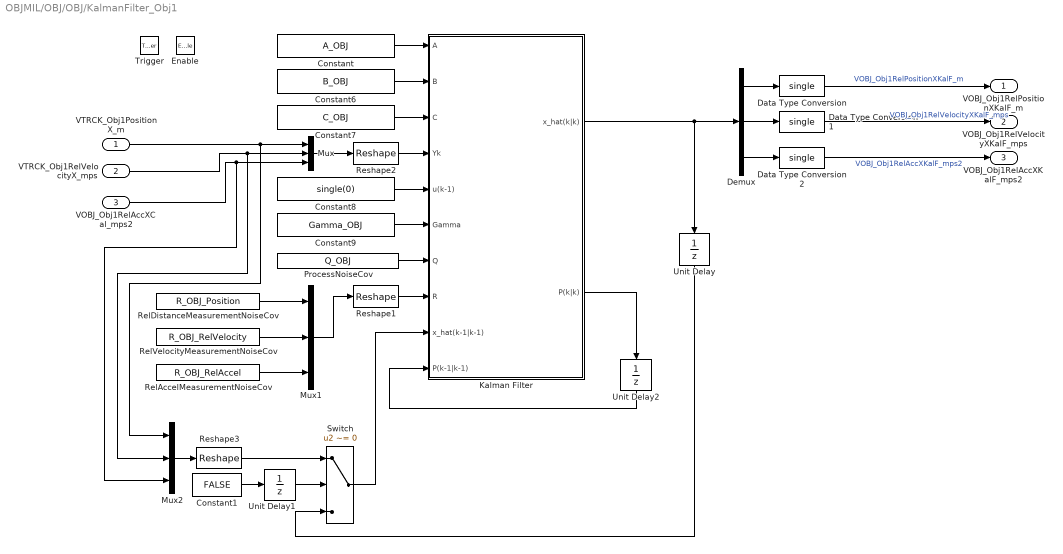
== system OBJMIL/OBJ/OBJ/KalmanFilter_Obj1 ==
  VTRCK_Obj1PositionX_m : Inport
  VTRCK_Obj1RelVelocityX_mps : Inport  Port=2
  VOBJ_Obj1RelAccXCal_mps2 : Inport  Port=3
  Enable : EnablePort  StatesWhenEnabling=reset
  Trigger : TriggerPort  PortDimensions=1
  Constant : Constant  Value=A_OBJ
  Constant1 : Constant  Value=FALSE
  Constant6 : Constant  Value=B_OBJ
  Constant7 : Constant  Value=C_OBJ
  Constant8 : Constant  Value=single(0)
  Constant9 : Constant  Value=Gamma_OBJ
  Data Type Conversion : DataTypeConversion  OutDataTypeStr=single
  Data Type Conversion1 : DataTypeConversion  OutDataTypeStr=single
  Data Type Conversion2 : DataTypeConversion  OutDataTypeStr=single
  Demux : Demux  Outputs=3
  Kalman Filter : Subsystem
  Mux : Mux  Inputs=3
  Mux1 : Mux  Inputs=3
  Mux2 : Mux  Inputs=3
  ProcessNoiseCov : Constant  Value=Q_OBJ
  RelAccelMeasurementNoiseCov : Constant  Value=R_OBJ_RelAccel  OutDataTypeStr=single
  RelDistanceMeasurementNoiseCov : Constant  Value=R_OBJ_Position  OutDataTypeStr=single
  RelVelocityMeasurementNoiseCov : Constant  Value=R_OBJ_RelVelocity  OutDataTypeStr=single
  Reshape1 : Reshape  OutputDimensionality=Customize  OutputDimensions=[3,3]
  Reshape2 : Reshape  OutputDimensionality=Customize  OutputDimensions=[3,1]
  Reshape3 : Reshape  OutputDimensionality=Customize  OutputDimensions=[3,1]
  Switch : Switch  Criteria=u2 ~= 0
  Unit Delay : UnitDelay  InitialCondition=single([0;0;0])  SampleTime=-1
  Unit Delay1 : UnitDelay  InitialCondition=TRUE  SampleTime=-1
  Unit Delay2 : UnitDelay  InitialCondition=single(eye(3,3))  SampleTime=-1
  VOBJ_Obj1RelPositionXKalF_m : Outport  OutputWhenDisabled=reset  InitialOutput=[0]
  VOBJ_Obj1RelVelocityXKalF_mps : Outport  Port=2  OutputWhenDisabled=reset  InitialOutput=[0]
  VOBJ_Obj1RelAccXKalF_mps2 : Outport  Port=3  OutputWhenDisabled=reset  InitialOutput=[0]
  wires:
  Data Type Conversion2/1 -> VOBJ_Obj1RelAccXKalF_mps2/1  "VOBJ_Obj1RelAccXKalF_mps2"
  Data Type Conversion1/1 -> VOBJ_Obj1RelVelocityXKalF_mps/1  "VOBJ_Obj1RelVelocityXKalF_mps"
  Data Type Conversion/1 -> VOBJ_Obj1RelPositionXKalF_m/1  "VOBJ_Obj1RelPositionXKalF_m"
  Kalman Filter/2(P(k|k)) -> Unit Delay2/1
  Unit Delay2/1 -> Kalman Filter/10(P(k-1|k-1))
  Kalman Filter/1(x_hat(k|k)) -> Unit Delay/1, Demux/1
  Unit Delay/1 -> Switch/3
  Constant9/1 -> Kalman Filter/6(Gamma)
  ProcessNoiseCov/1 -> Kalman Filter/7(Q)
  Mux1/1 -> Reshape1/1
  Reshape2/1 -> Kalman Filter/4(Yk)
  Mux/1 -> Reshape2/1
  Constant8/1 -> Kalman Filter/5(u(k-1))
  Constant/1 -> Kalman Filter/1(A)
  Constant6/1 -> Kalman Filter/2(B)
  Constant7/1 -> Kalman Filter/3(C)
  RelDistanceMeasurementNoiseCov/1 -> Mux1/1
  RelVelocityMeasurementNoiseCov/1 -> Mux1/2
  Reshape1/1 -> Kalman Filter/8(R)
  VTRCK_Obj1RelVelocityX_mps/1 -> Mux2/2, Mux/2
  VTRCK_Obj1PositionX_m/1 -> Mux2/1, Mux/1
  Demux/2 -> Data Type Conversion1/1
  Demux/1 -> Data Type Conversion/1
  Demux/3 -> Data Type Conversion2/1
  Constant1/1 -> Unit Delay1/1
  Unit Delay1/1 -> Switch/2
  VOBJ_Obj1RelAccXCal_mps2/1 -> Mux2/3, Mux/3
  Mux2/1 -> Reshape3/1
  Reshape3/1 -> Switch/1
  Switch/1 -> Kalman Filter/9(x_hat(k-1|k-1))
  RelAccelMeasurementNoiseCov/1 -> Mux1/3

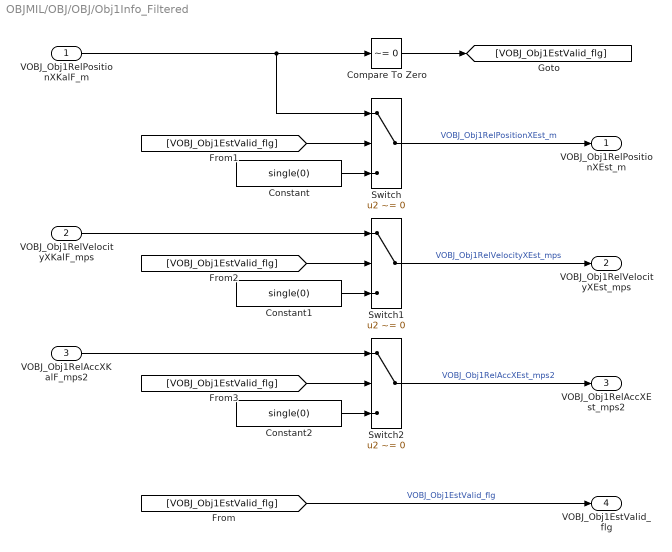
== system OBJMIL/OBJ/OBJ/Obj1Info_Filtered ==
  VOBJ_Obj1RelPositionXKalF_m : Inport
  VOBJ_Obj1RelVelocityXKalF_mps : Inport  Port=2
  VOBJ_Obj1RelAccXKalF_mps2 : Inport  Port=3
  Compare To Zero : simulink/Logic and Bit Operations/Compare To Zero  relop=~=  OutDataTypeStr=boolean
  Constant : Constant  Value=single(0)
  Constant1 : Constant  Value=single(0)
  Constant2 : Constant  Value=single(0)
  Switch : Switch  Criteria=u2 ~= 0
  Switch1 : Switch  Criteria=u2 ~= 0
  Switch2 : Switch  Criteria=u2 ~= 0
  VOBJ_Obj1RelPositionXEst_m : Outport
  VOBJ_Obj1RelVelocityXEst_mps : Outport  Port=2
  VOBJ_Obj1RelAccXEst_mps2 : Outport  Port=3
  VOBJ_Obj1EstValid_flg : Outport  Port=4
  wires:
  VOBJ_Obj1RelPositionXKalF_m/1 -> Switch/1, Compare To Zero/1
  Compare To Zero/1 -> [VOBJ_Obj1EstValid_flg]
  [VOBJ_Obj1EstValid_flg] -> VOBJ_Obj1EstValid_flg/1  "VOBJ_Obj1EstValid_flg"
  [VOBJ_Obj1EstValid_flg] -> Switch/2
  Switch/1 -> VOBJ_Obj1RelPositionXEst_m/1  "VOBJ_Obj1RelPositionXEst_m"
  Constant/1 -> Switch/3
  [VOBJ_Obj1EstValid_flg] -> Switch1/2
  Switch1/1 -> VOBJ_Obj1RelVelocityXEst_mps/1  "VOBJ_Obj1RelVelocityXEst_mps"
  Constant1/1 -> Switch1/3
  [VOBJ_Obj1EstValid_flg] -> Switch2/2
  Switch2/1 -> VOBJ_Obj1RelAccXEst_mps2/1  "VOBJ_Obj1RelAccXEst_mps2"
  Constant2/1 -> Switch2/3
  VOBJ_Obj1RelVelocityXKalF_mps/1 -> Switch1/1
  VOBJ_Obj1RelAccXKalF_mps2/1 -> Switch2/1

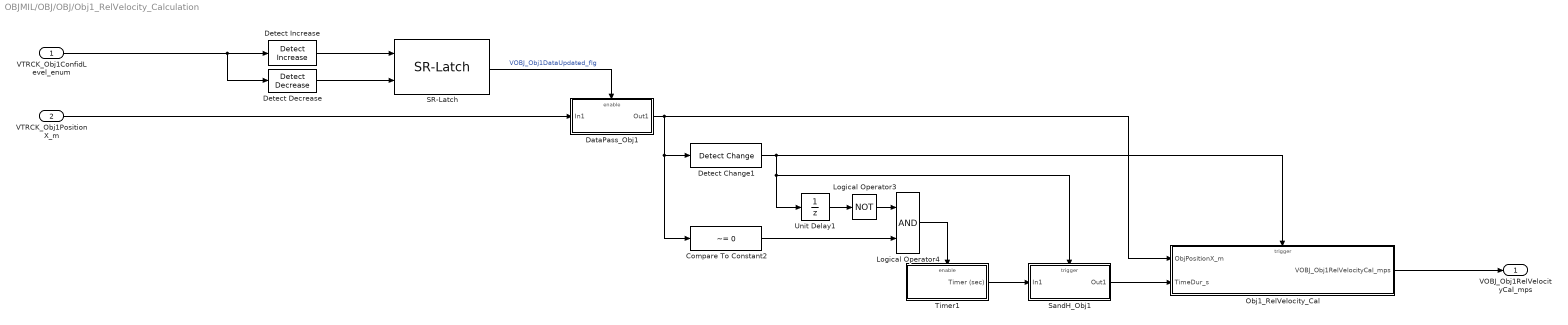
== system OBJMIL/OBJ/OBJ/Obj1_RelVelocity_Calculation ==
  VTRCK_Obj1ConfidLevel_enum : Inport
  VTRCK_Obj1PositionX_m : Inport  Port=2
  Compare To Constant2 : simulink/Logic and Bit Operations/Compare To Constant  relop=~=  const=0  OutDataTypeStr=boolean
  DataPass_Obj1 : Subsystem  TreatAsAtomicUnit=on
  Detect Change1 : simulink/Logic and Bit Operations/Detect Change  vinit=0  InputProcessing=Inherited  OutDataTypeStr=boolean
  Detect Decrease : simulink/Logic and Bit Operations/Detect Decrease  vinit=0.0  InputProcessing=Inherited  OutDataTypeStr=boolean
  Detect Increase : simulink/Logic and Bit Operations/Detect Increase  vinit=0.0  InputProcessing=Inherited  OutDataTypeStr=boolean
  Logical Operator3 : Logic  Operator=NOT  AllPortsSameDT=off  OutDataTypeStr=boolean
  Logical Operator4 : Logic  AllPortsSameDT=off  OutDataTypeStr=boolean
  Obj1_RelVelocity_Cal : Subsystem
  SR-Latch : hcu_lib/SR-Latch
  SandH_Obj1 : Subsystem  TreatAsAtomicUnit=on
  Timer1 : Subsystem  TreatAsAtomicUnit=on
  Unit Delay1 : UnitDelay  SampleTime=-1
  VOBJ_Obj1RelVelocityCal_mps : Outport
  wires:
  Obj1_RelVelocity_Cal/1(VOBJ_Obj1RelVelocityCal_mps) -> VOBJ_Obj1RelVelocityCal_mps/1
  Compare To Constant2/1 -> Logical Operator4/2
  Unit Delay1/1 -> Logical Operator3/1
  Logical Operator4/1 -> Timer1/Enable
  Logical Operator3/1 -> Logical Operator4/1
  SandH_Obj1/1(Out1) -> Obj1_RelVelocity_Cal/2(TimeDur_s)
  Timer1/1(Timer (sec)) -> SandH_Obj1/1(In1)
  DataPass_Obj1/1(Out1) -> Obj1_RelVelocity_Cal/1(ObjPositionX_m), Detect Change1/1, Compare To Constant2/1
  Detect Change1/1 -> Unit Delay1/1, SandH_Obj1/Trigger, Obj1_RelVelocity_Cal/Trigger
  VTRCK_Obj1PositionX_m/1 -> DataPass_Obj1/1(In1)
  SR-Latch/1 -> DataPass_Obj1/Enable  "VOBJ_Obj1DataUpdated_flg"
  Detect Increase/1 -> SR-Latch/1
  Detect Decrease/1 -> SR-Latch/2
  VTRCK_Obj1ConfidLevel_enum/1 -> Detect Decrease/1, Detect Increase/1

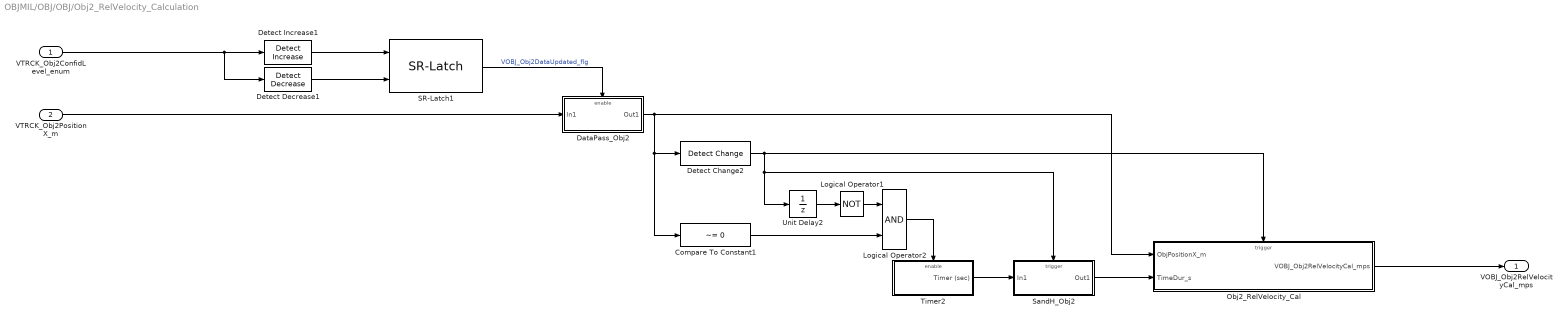
== system OBJMIL/OBJ/OBJ/Obj2_RelVelocity_Calculation ==
  VTRCK_Obj2ConfidLevel_enum : Inport
  VTRCK_Obj2PositionX_m : Inport  Port=2
  Compare To Constant1 : simulink/Logic and Bit Operations/Compare To Constant  relop=~=  const=0  OutDataTypeStr=boolean
  DataPass_Obj2 : Subsystem  TreatAsAtomicUnit=on
  Detect Change2 : simulink/Logic and Bit Operations/Detect Change  vinit=0  InputProcessing=Inherited  OutDataTypeStr=boolean
  Detect Decrease1 : simulink/Logic and Bit Operations/Detect Decrease  vinit=0.0  InputProcessing=Inherited  OutDataTypeStr=boolean
  Detect Increase1 : simulink/Logic and Bit Operations/Detect Increase  vinit=0.0  InputProcessing=Inherited  OutDataTypeStr=boolean
  Logical Operator1 : Logic  Operator=NOT  AllPortsSameDT=off  OutDataTypeStr=boolean
  Logical Operator2 : Logic  AllPortsSameDT=off  OutDataTypeStr=boolean
  Obj2_RelVelocity_Cal : Subsystem
  SR-Latch1 : hcu_lib/SR-Latch
  SandH_Obj2 : Subsystem  TreatAsAtomicUnit=on
  Timer2 : Subsystem  TreatAsAtomicUnit=on
  Unit Delay2 : UnitDelay  SampleTime=-1
  VOBJ_Obj2RelVelocityCal_mps : Outport
  wires:
  Detect Decrease1/1 -> SR-Latch1/2
  SR-Latch1/1 -> DataPass_Obj2/Enable  "VOBJ_Obj2DataUpdated_flg"
  Logical Operator2/1 -> Timer2/Enable
  SandH_Obj2/1(Out1) -> Obj2_RelVelocity_Cal/2(TimeDur_s)
  Compare To Constant1/1 -> Logical Operator2/2
  VTRCK_Obj2ConfidLevel_enum/1 -> Detect Increase1/1, Detect Decrease1/1
  VTRCK_Obj2PositionX_m/1 -> DataPass_Obj2/1(In1)
  Detect Change2/1 -> Obj2_RelVelocity_Cal/Trigger, SandH_Obj2/Trigger, Unit Delay2/1
  Detect Increase1/1 -> SR-Latch1/1
  DataPass_Obj2/1(Out1) -> Compare To Constant1/1, Detect Change2/1, Obj2_RelVelocity_Cal/1(ObjPositionX_m)
  Obj2_RelVelocity_Cal/1(VOBJ_Obj2RelVelocityCal_mps) -> VOBJ_Obj2RelVelocityCal_mps/1
  Logical Operator1/1 -> Logical Operator2/1
  Timer2/1(Timer (sec)) -> SandH_Obj2/1(In1)
  Unit Delay2/1 -> Logical Operator1/1

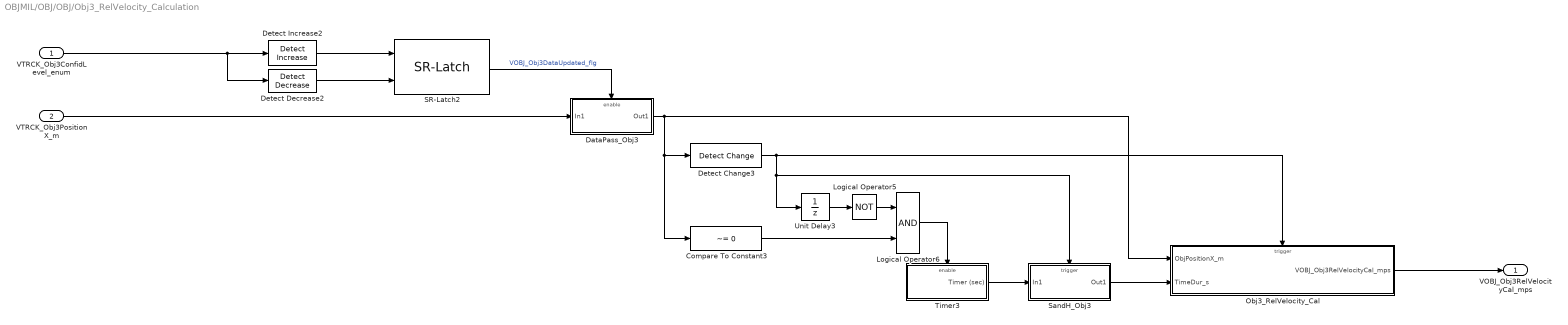
== system OBJMIL/OBJ/OBJ/Obj3_RelVelocity_Calculation ==
  VTRCK_Obj3ConfidLevel_enum : Inport
  VTRCK_Obj3PositionX_m : Inport  Port=2
  Compare To Constant3 : simulink/Logic and Bit Operations/Compare To Constant  relop=~=  const=0  OutDataTypeStr=boolean
  DataPass_Obj3 : Subsystem  TreatAsAtomicUnit=on
  Detect Change3 : simulink/Logic and Bit Operations/Detect Change  vinit=0  InputProcessing=Inherited  OutDataTypeStr=boolean
  Detect Decrease2 : simulink/Logic and Bit Operations/Detect Decrease  vinit=0.0  InputProcessing=Inherited  OutDataTypeStr=boolean
  Detect Increase2 : simulink/Logic and Bit Operations/Detect Increase  vinit=0.0  InputProcessing=Inherited  OutDataTypeStr=boolean
  Logical Operator5 : Logic  Operator=NOT  AllPortsSameDT=off  OutDataTypeStr=boolean
  Logical Operator6 : Logic  AllPortsSameDT=off  OutDataTypeStr=boolean
  Obj3_RelVelocity_Cal : Subsystem
  SR-Latch2 : hcu_lib/SR-Latch
  SandH_Obj3 : Subsystem  TreatAsAtomicUnit=on
  Timer3 : Subsystem  TreatAsAtomicUnit=on
  Unit Delay3 : UnitDelay  SampleTime=-1
  VOBJ_Obj3RelVelocityCal_mps : Outport
  wires:
  Detect Change3/1 -> Unit Delay3/1, SandH_Obj3/Trigger, Obj3_RelVelocity_Cal/Trigger
  Compare To Constant3/1 -> Logical Operator6/2
  Logical Operator5/1 -> Logical Operator6/1
  Detect Decrease2/1 -> SR-Latch2/2
  Obj3_RelVelocity_Cal/1(VOBJ_Obj3RelVelocityCal_mps) -> VOBJ_Obj3RelVelocityCal_mps/1
  VTRCK_Obj3ConfidLevel_enum/1 -> Detect Decrease2/1, Detect Increase2/1
  Timer3/1(Timer (sec)) -> SandH_Obj3/1(In1)
  SR-Latch2/1 -> DataPass_Obj3/Enable  "VOBJ_Obj3DataUpdated_flg"
  Detect Increase2/1 -> SR-Latch2/1
  Unit Delay3/1 -> Logical Operator5/1
  DataPass_Obj3/1(Out1) -> Obj3_RelVelocity_Cal/1(ObjPositionX_m), Detect Change3/1, Compare To Constant3/1
  VTRCK_Obj3PositionX_m/1 -> DataPass_Obj3/1(In1)
  SandH_Obj3/1(Out1) -> Obj3_RelVelocity_Cal/2(TimeDur_s)
  Logical Operator6/1 -> Timer3/Enable

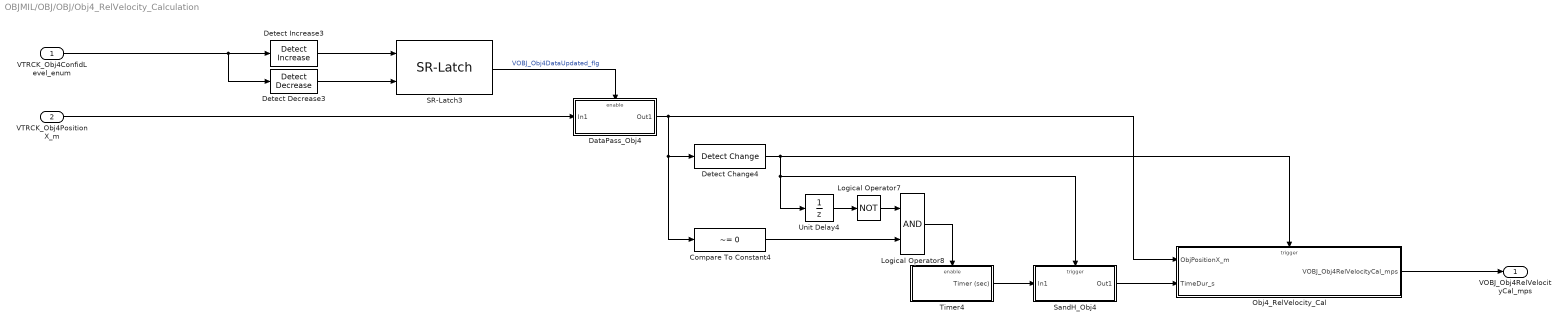
== system OBJMIL/OBJ/OBJ/Obj4_RelVelocity_Calculation ==
  VTRCK_Obj4ConfidLevel_enum : Inport
  VTRCK_Obj4PositionX_m : Inport  Port=2
  Compare To Constant4 : simulink/Logic and Bit Operations/Compare To Constant  relop=~=  const=0  OutDataTypeStr=boolean
  DataPass_Obj4 : Subsystem  TreatAsAtomicUnit=on
  Detect Change4 : simulink/Logic and Bit Operations/Detect Change  vinit=0  InputProcessing=Inherited  OutDataTypeStr=boolean
  Detect Decrease3 : simulink/Logic and Bit Operations/Detect Decrease  vinit=0.0  InputProcessing=Inherited  OutDataTypeStr=boolean
  Detect Increase3 : simulink/Logic and Bit Operations/Detect Increase  vinit=0.0  InputProcessing=Inherited  OutDataTypeStr=boolean
  Logical Operator7 : Logic  Operator=NOT  AllPortsSameDT=off  OutDataTypeStr=boolean
  Logical Operator8 : Logic  AllPortsSameDT=off  OutDataTypeStr=boolean
  Obj4_RelVelocity_Cal : Subsystem
  SR-Latch3 : hcu_lib/SR-Latch
  SandH_Obj4 : Subsystem  TreatAsAtomicUnit=on
  Timer4 : Subsystem  TreatAsAtomicUnit=on
  Unit Delay4 : UnitDelay  SampleTime=-1
  VOBJ_Obj4RelVelocityCal_mps : Outport
  wires:
  Logical Operator7/1 -> Logical Operator8/1
  Compare To Constant4/1 -> Logical Operator8/2
  Timer4/1(Timer (sec)) -> SandH_Obj4/1(In1)
  Logical Operator8/1 -> Timer4/Enable
  SandH_Obj4/1(Out1) -> Obj4_RelVelocity_Cal/2(TimeDur_s)
  Unit Delay4/1 -> Logical Operator7/1
  Obj4_RelVelocity_Cal/1(VOBJ_Obj4RelVelocityCal_mps) -> VOBJ_Obj4RelVelocityCal_mps/1
  Detect Change4/1 -> Obj4_RelVelocity_Cal/Trigger, SandH_Obj4/Trigger, Unit Delay4/1
  DataPass_Obj4/1(Out1) -> Compare To Constant4/1, Detect Change4/1, Obj4_RelVelocity_Cal/1(ObjPositionX_m)
  Detect Increase3/1 -> SR-Latch3/1
  VTRCK_Obj4ConfidLevel_enum/1 -> Detect Increase3/1, Detect Decrease3/1
  SR-Latch3/1 -> DataPass_Obj4/Enable  "VOBJ_Obj4DataUpdated_flg"
  VTRCK_Obj4PositionX_m/1 -> DataPass_Obj4/1(In1)
  Detect Decrease3/1 -> SR-Latch3/2

== system OBJMIL/OBJ/OBJ/Obj5_RelVelocity_Calculation ==
  VTRCK_Obj5ConfidLevel_enum : Inport
  VTRCK_Obj5PositionX_m : Inport  Port=2
  Compare To Constant5 : simulink/Logic and Bit Operations/Compare To Constant  relop=~=  const=0  OutDataTypeStr=boolean
  DataPass_Obj5 : Subsystem  TreatAsAtomicUnit=on
  Detect Change5 : simulink/Logic and Bit Operations/Detect Change  vinit=0  InputProcessing=Inherited  OutDataTypeStr=boolean
  Detect Decrease4 : simulink/Logic and Bit Operations/Detect Decrease  vinit=0.0  InputProcessing=Inherited  OutDataTypeStr=boolean
  Detect Increase4 : simulink/Logic and Bit Operations/Detect Increase  vinit=0.0  InputProcessing=Inherited  OutDataTypeStr=boolean
  Logical Operator10 : Logic  AllPortsSameDT=off  OutDataTypeStr=boolean
  Logical Operator9 : Logic  Operator=NOT  AllPortsSameDT=off  OutDataTypeStr=boolean
  Obj5_RelVelocity_Cal : Subsystem
  SR-Latch4 : hcu_lib/SR-Latch
  SandH_Obj5 : Subsystem  TreatAsAtomicUnit=on
  Timer5 : Subsystem  TreatAsAtomicUnit=on
  Unit Delay5 : UnitDelay  SampleTime=-1
  VOBJ_Obj5RelVelocityCal_mps : Outport
  wires:
  Obj5_RelVelocity_Cal/1(VOBJ_Obj5RelVelocityCal_mps) -> VOBJ_Obj5RelVelocityCal_mps/1
  Unit Delay5/1 -> Logical Operator9/1
  Compare To Constant5/1 -> Logical Operator10/2
  Logical Operator10/1 -> Timer5/Enable
  Logical Operator9/1 -> Logical Operator10/1
  SandH_Obj5/1(Out1) -> Obj5_RelVelocity_Cal/2(TimeDur_s)
  Timer5/1(Timer (sec)) -> SandH_Obj5/1(In1)
  Detect Decrease4/1 -> SR-Latch4/2
  Detect Increase4/1 -> SR-Latch4/1
  VTRCK_Obj5ConfidLevel_enum/1 -> Detect Decrease4/1, Detect Increase4/1
  Detect Change5/1 -> Unit Delay5/1, SandH_Obj5/Trigger, Obj5_RelVelocity_Cal/Trigger
  DataPass_Obj5/1(Out1) -> Obj5_RelVelocity_Cal/1(ObjPositionX_m), Detect Change5/1, Compare To Constant5/1
  SR-Latch4/1 -> DataPass_Obj5/Enable  "VOBJ_Obj5DataUpdated_flg"
  VTRCK_Obj5PositionX_m/1 -> DataPass_Obj5/1(In1)

== system OBJMIL/OBJ/OBJ/Trigger signal generator ==
  Constant3 : Constant  Value=KOBJ_KalmanFilterCalRate_s
  trigger signal generator : Subsystem  TreatAsAtomicUnit=on
  Trigger_signal : Outport
  wires:
  trigger signal generator/1(Trigger_signal) -> Trigger_signal/1
  Constant3/1 -> trigger signal generator/1(Time_dur [s])

== system OBJMIL/OBJ/OBJ/Trigger signal generator1 ==
  Constant3 : Constant  Value=KOBJ_VehAccCalRate_s
  trigger signal generator : Subsystem  TreatAsAtomicUnit=on
  Trigger_signal : Outport
  wires:
  trigger signal generator/1(Trigger_signal) -> Trigger_signal/1
  Constant3/1 -> trigger signal generator/1(Time_dur [s])

== system OBJMIL/OBJ/OBJ/Vehicle Acceleration Calculation ==
  note: m/s^2
  note: m/s
  note: km/h
  In1 : Inport
  Trigger : TriggerPort
  Constant2 : Constant  Value=KOBJ_VehAccCalRate_s
  Constant3 : Constant  Value=KOBJ_VehAccCalRate_s
  Constant4 : Constant  Value=KOBJ_VehAccFltConst_s
  Divide : Product  Inputs=*/
  Gain : Gain  Gain=1000/3600
  Sum : Sum  Inputs=+-
  Unit Delay : UnitDelay  SampleTime=-1
  signal_filter : Subsystem
  VOBJ_VehAcc_mps2 : Outport
  wires:
  signal_filter/1(raw_input_filt) -> VOBJ_VehAcc_mps2/1  "VOBJ_VehAcc_mps2"
  Constant3/1 -> Divide/2
  Gain/1 -> Divide/1
  Sum/1 -> Gain/1
  Unit Delay/1 -> Sum/2
  In1/1 -> Sum/1, Unit Delay/1
  Constant2/1 -> signal_filter/3(Ts)
  Constant4/1 -> signal_filter/2(Tc)
  Divide/1 -> signal_filter/1(raw_input)  "VOBJ_VehAcclUnFlt_mps2"

== system OBJMIL/OBJ/model_info/EmptySubsystem ==

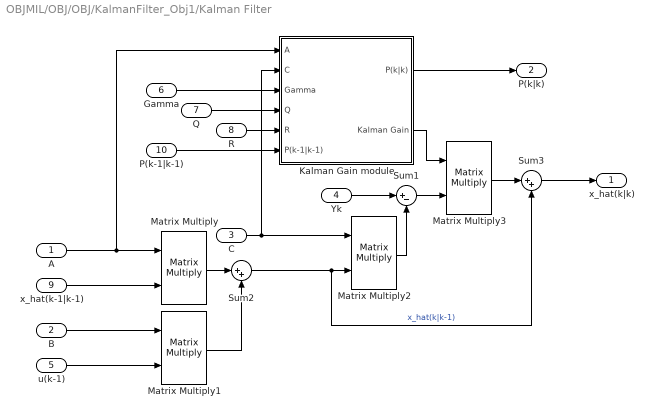
== system OBJMIL/OBJ/OBJ/KalmanFilter_Obj1/Kalman Filter ==
  A : Inport
  B : Inport  Port=2
  C : Inport  Port=3
  Yk : Inport  Port=4
  u(k-1) : Inport  Port=5
  Gamma : Inport  Port=6
  Q : Inport  Port=7
  R : Inport  Port=8
  x_hat(k-1|k-1) : Inport  Port=9
  P(k-1|k-1) : Inport  Port=10
  Kalman Gain module : Subsystem
  Matrix Multiply{,1..3} (4 alike) : Product  Multiplication=Matrix(*)
  Sum1 : Sum  Inputs=|+-
  Sum2 : Sum  Inputs=|++
  Sum3 : Sum  Inputs=|++
  x_hat(k|k) : Outport
  P(k|k) : Outport  Port=2
  wires:
  A/1 -> Matrix Multiply/1, Kalman Gain module/1(A)
  x_hat(k-1|k-1)/1 -> Matrix Multiply/2
  Matrix Multiply/1 -> Sum2/1
  B/1 -> Matrix Multiply1/1
  u(k-1)/1 -> Matrix Multiply1/2
  Matrix Multiply1/1 -> Sum2/2
  Yk/1 -> Sum1/1
  C/1 -> Matrix Multiply2/1, Kalman Gain module/2(C)
  Sum2/1 -> Matrix Multiply2/2, Sum3/2  "x_hat(k|k-1)"
  Matrix Multiply2/1 -> Sum1/2
  Kalman Gain module/2(Kalman Gain) -> Matrix Multiply3/1
  Sum1/1 -> Matrix Multiply3/2
  Matrix Multiply3/1 -> Sum3/1
  Sum3/1 -> x_hat(k|k)/1
  Gamma/1 -> Kalman Gain module/3(Gamma)
  Q/1 -> Kalman Gain module/4(Q)
  R/1 -> Kalman Gain module/5(R)
  Kalman Gain module/1(P(k|k)) -> P(k|k)/1
  P(k-1|k-1)/1 -> Kalman Gain module/6(P(k-1|k-1))

== system OBJMIL/OBJ/OBJ/Obj1_RelVelocity_Calculation/DataPass_Obj1 ==
  In1 : Inport
  Enable : EnablePort  StatesWhenEnabling=reset
  Out1 : Outport  OutputWhenDisabled=reset  InitialOutput=[0]
  wires:
  In1/1 -> Out1/1

== system OBJMIL/OBJ/OBJ/Obj1_RelVelocity_Calculation/Obj1_RelVelocity_Cal ==
  ObjPositionX_m : Inport
  TimeDur_s : Inport  Port=2
  Trigger : TriggerPort
  Compare To Zero1 : simulink/Logic and Bit Operations/Compare To Zero  relop=~=  OutDataTypeStr=boolean
  Compare To Zero2 : simulink/Logic and Bit Operations/Compare To Zero  relop=~=  OutDataTypeStr=boolean
  Compare To Zero3 : simulink/Logic and Bit Operations/Compare To Zero  relop=~=  OutDataTypeStr=boolean
  Constant1 : Constant  Value=0  OutDataTypeStr=single
  Enabled Subsystem : Subsystem  TreatAsAtomicUnit=on
  Logical Operator : Logic  Inputs=3  AllPortsSameDT=off  OutDataTypeStr=boolean
  Sum : Sum  Inputs=+-
  Unit Delay : UnitDelay  SampleTime=-1
  Unit Delay2 : UnitDelay  SampleTime=-1
  divide : hcu_lib/divide
  VOBJ_Obj1RelVelocityCal_mps : Outport
  wires:
  Unit Delay2/1 -> Compare To Zero3/1
  Compare To Zero3/1 -> Logical Operator/3
  Enabled Subsystem/1(Out1) -> divide/1
  Sum/1 -> Enabled Subsystem/1(In1)
  Logical Operator/1 -> Enabled Subsystem/Enable
  Compare To Zero2/1 -> Logical Operator/2
  Compare To Zero1/1 -> Logical Operator/1
  Constant1/1 -> divide/3
  TimeDur_s/1 -> divide/2
  ObjPositionX_m/1 -> Unit Delay/1, Sum/1, Compare To Zero1/1
  Unit Delay/1 -> Sum/2, Unit Delay2/1, Compare To Zero2/1
  divide/1 -> VOBJ_Obj1RelVelocityCal_mps/1  "VOBJ_Obj1RelVelocityCal_mps"

== system OBJMIL/OBJ/OBJ/Obj1_RelVelocity_Calculation/SandH_Obj1 ==
  In1 : Inport
  Trigger : TriggerPort
  Out1 : Outport
  wires:
  In1/1 -> Out1/1

== system OBJMIL/OBJ/OBJ/Obj1_RelVelocity_Calculation/Timer1 ==
  Enable : EnablePort  StatesWhenEnabling=reset  ZeroCross=off
  Constant : Constant  Value=C_TASK_5MS_S
  Sum : Sum  Inputs=|++  SaturateOnIntegerOverflow=on  InputSameDT=on
  Unit Delay : UnitDelay  SampleTime=-1
  Timer (sec) : Outport  OutputWhenDisabled=reset  InitialOutput=0
  wires:
  Constant/1 -> Sum/1
  Sum/1 -> Unit Delay/1
  Unit Delay/1 -> Sum/2, Timer (sec)/1

== system OBJMIL/OBJ/OBJ/Obj2_RelVelocity_Calculation/DataPass_Obj2 ==
  In1 : Inport
  Enable : EnablePort  StatesWhenEnabling=reset
  Out1 : Outport  OutputWhenDisabled=reset  InitialOutput=[0]
  wires:
  In1/1 -> Out1/1

== system OBJMIL/OBJ/OBJ/Obj2_RelVelocity_Calculation/Obj2_RelVelocity_Cal ==
  ObjPositionX_m : Inport
  TimeDur_s : Inport  Port=2
  Trigger : TriggerPort
  Compare To Zero1 : simulink/Logic and Bit Operations/Compare To Zero  relop=~=  OutDataTypeStr=boolean
  Compare To Zero2 : simulink/Logic and Bit Operations/Compare To Zero  relop=~=  OutDataTypeStr=boolean
  Compare To Zero3 : simulink/Logic and Bit Operations/Compare To Zero  relop=~=  OutDataTypeStr=boolean
  Constant1 : Constant  Value=0  OutDataTypeStr=single
  Enabled Subsystem : Subsystem  TreatAsAtomicUnit=on
  Logical Operator : Logic  Inputs=3  AllPortsSameDT=off  OutDataTypeStr=boolean
  Sum : Sum  Inputs=+-
  Unit Delay : UnitDelay  SampleTime=-1
  Unit Delay2 : UnitDelay  SampleTime=-1
  divide : hcu_lib/divide
  VOBJ_Obj2RelVelocityCal_mps : Outport
  wires:
  divide/1 -> VOBJ_Obj2RelVelocityCal_mps/1  "VOBJ_Obj2RelVelocityCal_mps"
  Unit Delay/1 -> Compare To Zero2/1, Unit Delay2/1, Sum/2
  ObjPositionX_m/1 -> Compare To Zero1/1, Sum/1, Unit Delay/1
  TimeDur_s/1 -> divide/2
  Constant1/1 -> divide/3
  Compare To Zero1/1 -> Logical Operator/1
  Compare To Zero2/1 -> Logical Operator/2
  Logical Operator/1 -> Enabled Subsystem/Enable
  Sum/1 -> Enabled Subsystem/1(In1)
  Enabled Subsystem/1(Out1) -> divide/1
  Compare To Zero3/1 -> Logical Operator/3
  Unit Delay2/1 -> Compare To Zero3/1

== system OBJMIL/OBJ/OBJ/Obj2_RelVelocity_Calculation/SandH_Obj2 ==
  In1 : Inport
  Trigger : TriggerPort
  Out1 : Outport
  wires:
  In1/1 -> Out1/1

== system OBJMIL/OBJ/OBJ/Obj2_RelVelocity_Calculation/Timer2 ==
  Enable : EnablePort  StatesWhenEnabling=reset  ZeroCross=off
  Constant : Constant  Value=C_TASK_5MS_S
  Sum : Sum  Inputs=|++  SaturateOnIntegerOverflow=on  InputSameDT=on
  Unit Delay : UnitDelay  SampleTime=-1
  Timer (sec) : Outport  OutputWhenDisabled=reset  InitialOutput=0
  wires:
  Unit Delay/1 -> Timer (sec)/1, Sum/2
  Sum/1 -> Unit Delay/1
  Constant/1 -> Sum/1

== system OBJMIL/OBJ/OBJ/Obj3_RelVelocity_Calculation/DataPass_Obj3 ==
  In1 : Inport
  Enable : EnablePort  StatesWhenEnabling=reset
  Out1 : Outport  OutputWhenDisabled=reset  InitialOutput=[0]
  wires:
  In1/1 -> Out1/1

== system OBJMIL/OBJ/OBJ/Obj3_RelVelocity_Calculation/Obj3_RelVelocity_Cal ==
  ObjPositionX_m : Inport
  TimeDur_s : Inport  Port=2
  Trigger : TriggerPort
  Compare To Zero1 : simulink/Logic and Bit Operations/Compare To Zero  relop=~=  OutDataTypeStr=boolean
  Compare To Zero2 : simulink/Logic and Bit Operations/Compare To Zero  relop=~=  OutDataTypeStr=boolean
  Compare To Zero3 : simulink/Logic and Bit Operations/Compare To Zero  relop=~=  OutDataTypeStr=boolean
  Constant1 : Constant  Value=0  OutDataTypeStr=single
  Enabled Subsystem : Subsystem  TreatAsAtomicUnit=on
  Logical Operator : Logic  Inputs=3  AllPortsSameDT=off  OutDataTypeStr=boolean
  Sum : Sum  Inputs=+-
  Unit Delay : UnitDelay  SampleTime=-1
  Unit Delay2 : UnitDelay  SampleTime=-1
  divide : hcu_lib/divide
  VOBJ_Obj3RelVelocityCal_mps : Outport
  wires:
  Unit Delay2/1 -> Compare To Zero3/1
  Compare To Zero3/1 -> Logical Operator/3
  Enabled Subsystem/1(Out1) -> divide/1
  Sum/1 -> Enabled Subsystem/1(In1)
  Logical Operator/1 -> Enabled Subsystem/Enable
  Compare To Zero2/1 -> Logical Operator/2
  Compare To Zero1/1 -> Logical Operator/1
  Constant1/1 -> divide/3
  TimeDur_s/1 -> divide/2
  ObjPositionX_m/1 -> Unit Delay/1, Sum/1, Compare To Zero1/1
  Unit Delay/1 -> Sum/2, Unit Delay2/1, Compare To Zero2/1
  divide/1 -> VOBJ_Obj3RelVelocityCal_mps/1  "VOBJ_Obj3RelVelocityCal_mps"

== system OBJMIL/OBJ/OBJ/Obj3_RelVelocity_Calculation/SandH_Obj3 ==
  In1 : Inport
  Trigger : TriggerPort
  Out1 : Outport
  wires:
  In1/1 -> Out1/1

== system OBJMIL/OBJ/OBJ/Obj3_RelVelocity_Calculation/Timer3 ==
  Enable : EnablePort  StatesWhenEnabling=reset  ZeroCross=off
  Constant : Constant  Value=C_TASK_5MS_S
  Sum : Sum  Inputs=|++  SaturateOnIntegerOverflow=on  InputSameDT=on
  Unit Delay : UnitDelay  SampleTime=-1
  Timer (sec) : Outport  OutputWhenDisabled=reset  InitialOutput=0
  wires:
  Constant/1 -> Sum/1
  Sum/1 -> Unit Delay/1
  Unit Delay/1 -> Sum/2, Timer (sec)/1

== system OBJMIL/OBJ/OBJ/Obj4_RelVelocity_Calculation/DataPass_Obj4 ==
  In1 : Inport
  Enable : EnablePort  StatesWhenEnabling=reset
  Out1 : Outport  OutputWhenDisabled=reset  InitialOutput=[0]
  wires:
  In1/1 -> Out1/1
